simulink model "chap5_11sim"  (Simulink 6.3)
settings: Solver=ode45  StartTime=0.0  StopTime=50  FixedStep=0.001  RelTol=1e-3  AbsTol=1e-3
settings Model: LastModifiedBy=Administrator  ExtModeTrigMode=oneshot  ExtModeArmWhenConnect=off  StrictBusMsg=None
settings DataIOCC: LimitDataPoints=off  SignalLoggingName=sigsOut
settings OptimizationCC: BooleanDataType=off
settings DebuggingCC: SolverPrmCheckMsg=none
settings HardwareCC: TargetUnknown=on

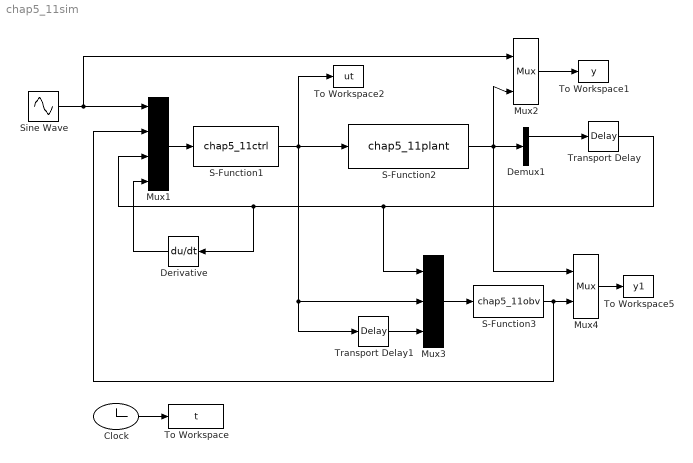
== system chap5_11sim ==
  Clock : Clock
  Demux1 : Demux  Outputs=2
  Derivative : Derivative  Orientation=left
  Mux1 : Mux
  Mux2 : Mux  Inputs=2
  Mux3 : Mux  Inputs=3
  Mux4 : Mux  Inputs=2
  S-Function1 : S-Function  FunctionName=chap5_11ctrl
  S-Function2 : S-Function  FunctionName=chap5_11plant
  S-Function3 : S-Function  FunctionName=chap5_11obv
  Sine Wave : Sin  SampleTime=0
  To Workspace : ToWorkspace  VariableName=t  SampleTime=-1  SaveFormat=Array
  To Workspace1 : ToWorkspace  VariableName=y  SampleTime=-1  SaveFormat=Array
  To Workspace2 : ToWorkspace  VariableName=ut  SampleTime=-1  SaveFormat=Array
  To Workspace5 : ToWorkspace  VariableName=y1  SampleTime=-1  SaveFormat=Array
  Transport Delay : TransportDelay  DelayTime=3
  Transport Delay1 : TransportDelay  DelayTime=3
  wires:
  Clock/1 -> To Workspace/1
  Mux3/1 -> S-Function3/1
  Transport Delay1/1 -> Mux3/3
  S-Function2/1 -> Demux1/1, Mux4/1, Mux2/2
  Demux1/1 -> Transport Delay/1
  Transport Delay/1 -> Mux3/1, Mux1/3, Derivative/1
  Mux2/1 -> To Workspace1/1
  Mux4/1 -> To Workspace5/1
  S-Function3/1 -> Mux4/2, Mux1/2
  S-Function1/1 -> S-Function2/1, To Workspace2/1, Mux3/2, Transport Delay1/1
  Mux1/1 -> S-Function1/1
  Sine Wave/1 -> Mux1/1, Mux2/1
  Derivative/1 -> Mux1/4
